simulink model "beb_ut"  (Simulink 8.1)
settings: Solver=ode45  StartTime=0.0  StopTime=10.0  RelTol=1e-3
libraries: siltestlib x6, beb x1
settings Model: Creator=xsellart  LastModifiedBy=AT015411
settings DataIOCC: SignalLoggingSaveFormat=Dataset
settings OptimizationCC: ExpressionDepthLimit=128
settings DebuggingCC: FcnCallInpInsideContextMsg=EnableAllAsError
settings GRTTargetCC: CombineOutputUpdateFcns=on  GRTInterface=off

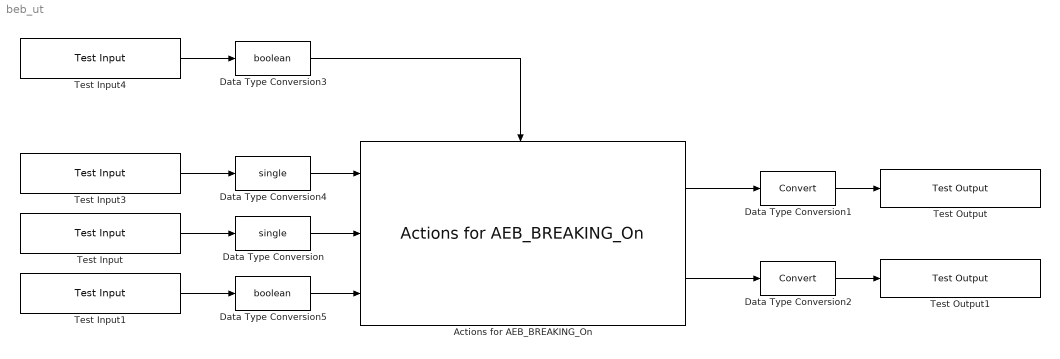
== system beb_ut ==
  Actions for AEB_BREAKING_On : beb/Actions for AEB_BREAKING_On
  Data Type Conversion : DataTypeConversion  OutDataTypeStr=single
  Data Type Conversion1 : DataTypeConversion
  Data Type Conversion2 : DataTypeConversion
  Data Type Conversion3 : DataTypeConversion  OutDataTypeStr=boolean
  Data Type Conversion4 : DataTypeConversion  OutDataTypeStr=single
  Data Type Conversion5 : DataTypeConversion  OutDataTypeStr=boolean
  Test Input : siltestlib/Test Input  varname=VDINR_VehSpd_mps  sampletime=-1
  Test Input1 : siltestlib/Test Input  varname=VAEB_AEBReq_flg  sampletime=-1
  Test Input3 : siltestlib/Test Input  varname=VAEB_AEBDecelReq_mps2  sampletime=-1
  Test Input4 : siltestlib/Test Input  varname=VAEB_AEBActing_flg  sampletime=-1
  Test Output : siltestlib/Test Output  varname=VAEB_WarningLightsReq_flg  sampletime=-1
  Test Output1 : siltestlib/Test Output  varname=VAEB_AEBHoldReq_flg  sampletime=-1
  wires:
  Test Input/1 -> Data Type Conversion/1
  Data Type Conversion/1 -> Actions for AEB_BREAKING_On/2
  Test Input3/1 -> Data Type Conversion4/1
  Test Input4/1 -> Data Type Conversion3/1
  Data Type Conversion3/1 -> Actions for AEB_BREAKING_On/Enable
  Data Type Conversion4/1 -> Actions for AEB_BREAKING_On/1
  Test Input1/1 -> Data Type Conversion5/1
  Data Type Conversion5/1 -> Actions for AEB_BREAKING_On/3
  Actions for AEB_BREAKING_On/1 -> Data Type Conversion1/1
  Actions for AEB_BREAKING_On/2 -> Data Type Conversion2/1
  Data Type Conversion1/1 -> Test Output/1
  Data Type Conversion2/1 -> Test Output1/1
